simulink model "class_6_simulink"  (R2023b)
settings: Solver=VariableStepAuto  StartTime=0.0  StopTime=Tsim  RelTol=1e-3
values from neighbouring files (symbols this model uses):
  finaldisturbancevalue = 1    [class_6.m]
  h = 6.5    [class_6.m]
  initialdisturbancevalue = 0    [class_6.m]
  Tdisturbance = 8    [class_6.m]
  Ts = 0.5    [class_6.m]
libraries: cstblocks x7
settings Model: Creator=klysm  LastModifiedBy=klysm

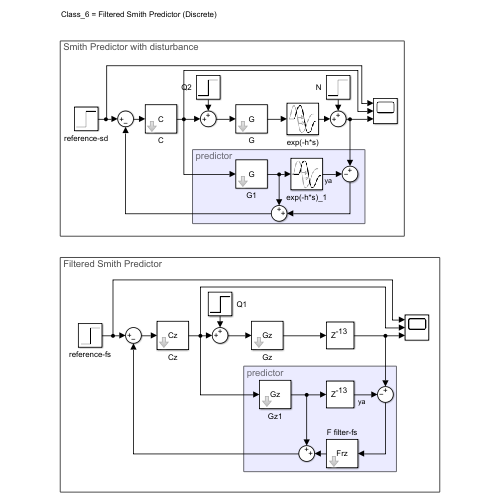
[thumbnail: Simulink's stored preview of the top-level diagram]
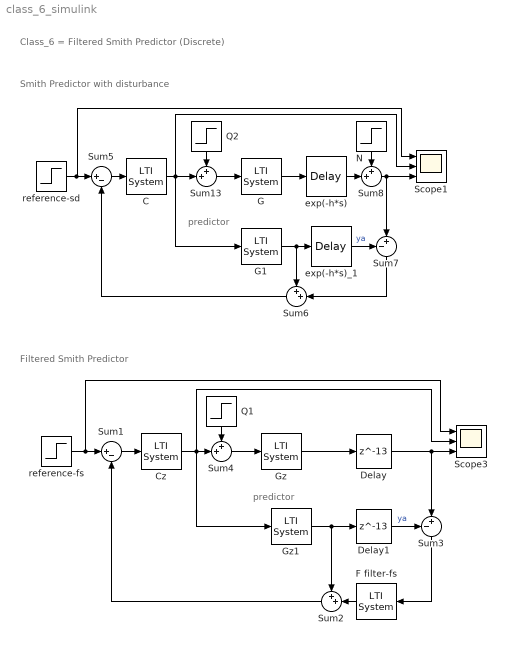
== system class_6_simulink ==
  note: Class_6 = Filtered Smith Predictor (Discrete)
  note: Filtered Smith Predictor
  note: predictor
  note: predictor
  note: Smith Predictor with disturbance
  C : cstblocks/LTI System  sys=C  IC=[]  PadeOrder=0
  Cz : cstblocks/LTI System  sys=Cz  IC=[]  PadeOrder=0
  Delay : Delay  DelayLength=13  SampleTime=Ts
  Delay1 : Delay  DelayLength=13  SampleTime=Ts
  F filter-fs : cstblocks/LTI System  sys=Frz  IC=[]  PadeOrder=0
  G : cstblocks/LTI System  sys=G  IC=[]  PadeOrder=0
  G1 : cstblocks/LTI System  sys=G  IC=[]  PadeOrder=0
  Gz : cstblocks/LTI System  sys=Gz  IC=[]  PadeOrder=0
  Gz1 : cstblocks/LTI System  sys=Gz  IC=[]  PadeOrder=0
  N : Step  Time=20  After=0.2  SampleTime=0
  Q1 : Step  Time=Tdisturbance  Before=initialdisturbancevalue  After=finaldisturbancevalue  SampleTime=0
  Q2 : Step  Time=10  After=0.2  SampleTime=0
  Scope1 : Scope  NumInputPorts=3
  Scope3 : Scope  NumInputPorts=3
  Sum1 : Sum  Inputs=|+-
  Sum{2,4,6,8,13} (5 alike) : Sum  Inputs=++|
  Sum3 : Sum  Inputs=-+|
  Sum5 : Sum  Inputs=|+-
  Sum7 : Sum  Inputs=-+|
  exp(-h*s) : TransportDelay  DelayTime=h
  exp(-h*s)_1 : TransportDelay  DelayTime=h
  reference-fs : Step  SampleTime=0
  reference-sd : Step  Time=0  SampleTime=0
  wires:
  Sum3/1 -> F filter-fs/1
  reference-fs/1 -> Scope3/1, Sum1/1
  Gz1/1 -> Delay1/1, Sum2/1
  Gz/1 -> Delay/1
  Sum2/1 -> Sum1/2
  Delay1/1 -> Sum3/1  "ya"
  Sum4/1 -> Gz/1
  Delay/1 -> Scope3/3, Sum3/2
  Sum1/1 -> Cz/1
  Q1/1 -> Sum4/1
  F filter-fs/1 -> Sum2/2
  Cz/1 -> Gz1/1, Scope3/2, Sum4/2
  Q2/1 -> Sum13/1
  Sum13/1 -> G/1
  Sum5/1 -> C/1
  N/1 -> Sum8/1
  Sum8/1 -> Scope1/3, Sum7/2
  exp(-h*s)_1/1 -> Sum7/1  "ya"
  G1/1 -> Sum6/1, exp(-h*s)_1/1
  Sum6/1 -> Sum5/2
  Sum7/1 -> Sum6/2
  reference-sd/1 -> Scope1/1, Sum5/1
  exp(-h*s)/1 -> Sum8/2
  G/1 -> exp(-h*s)/1
  C/1 -> G1/1, Sum13/2, Scope1/2
